simulink model "bergman_otro_modelo"  (R2019b)
settings: Solver=VariableStepAuto  StartTime=0.0  StopTime=86400  RelTol=1e-3
undefined symbols (not defined in the file): n, p1, p2, p3, Vi
libraries: simulink x16
settings Model: Creator=USUARIO  LastModifiedBy=USUARIO

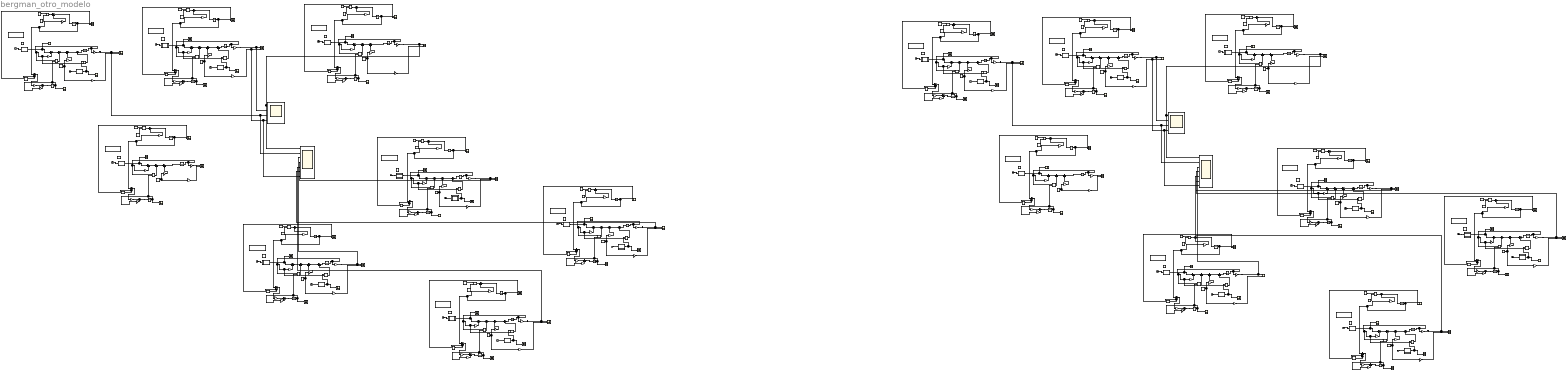
== system bergman_otro_modelo ==
  Clock{1..28} (28 alike) : Clock
  Constant{1,3,5,7,9,11,13,15,17,19,21,24,26,28,30,32} (16 alike) : Constant  Value=0
  Constant{2,4,6,8,10,12,14,16,18,20,22..23,25,27,29,31} (16 alike) : Constant  Value=Vi
  Divide{1..16} (16 alike) : Product  Inputs=*/
  Gain{1,6,11,13,18,20,25,27,32,34,39,41,46,48,50,52,54,59,62,67..68,73,76,82,84,89,92,97,99,102..103,109} (32 alike) : Gain  Gain=p1
  Gain{3,5,8,10,15,17,22,24,29,31,36,38,43,45,51,56,58,64,66,70,72,78..79,81,86,88,94,96,101,106,108,111} (32 alike) : Gain  Gain=18
  Gain{2,14,21,28,35,42,49,55,61,63,69,77,85,93,100,104} (16 alike) : Gain  Gain=p3
  Gain{7,12,19,26,33,40,47,53,60,74..75,83,91,98,105,110} (16 alike) : Gain  Gain=p2
  Gain{4,9,16,23,30,37,44,57,65,71,80,87,90,95,107,112} (16 alike) : Gain  Gain=n
  Glucosa basal{1..16} (16 alike) : Constant  Value=7
  Grafica ingesta D{1..28} (28 alike) : Scope
  Ingesta 75 g1 : MATLAB Function  TreatAsAtomicUnit=on
  Ingesta 75 g10 : MATLAB Function  TreatAsAtomicUnit=on
  Ingesta 75 g11 : MATLAB Function  TreatAsAtomicUnit=on
  Ingesta 75 g12 : MATLAB Function  TreatAsAtomicUnit=on
  Ingesta 75 g13 : MATLAB Function  TreatAsAtomicUnit=on
  Ingesta 75 g14 : MATLAB Function  TreatAsAtomicUnit=on
  Ingesta 75 g15 : MATLAB Function  TreatAsAtomicUnit=on
  Ingesta 75 g16 : MATLAB Function  TreatAsAtomicUnit=on
  Ingesta 75 g2 : MATLAB Function  TreatAsAtomicUnit=on
  Ingesta 75 g3 : MATLAB Function  TreatAsAtomicUnit=on
  Ingesta 75 g4 : MATLAB Function  TreatAsAtomicUnit=on
  Ingesta 75 g5 : MATLAB Function  TreatAsAtomicUnit=on
  Ingesta 75 g6 : MATLAB Function  TreatAsAtomicUnit=on
  Ingesta 75 g7 : MATLAB Function  TreatAsAtomicUnit=on
  Ingesta 75 g8 : MATLAB Function  TreatAsAtomicUnit=on
  Ingesta 75 g9 : MATLAB Function  TreatAsAtomicUnit=on
  Insulina basal{1..16} (16 alike) : Constant  Value=10
  Integrator{1,4,7,10,13,16,19} (7 alike) : Integrator  InitialCondition=10
  Integrator{2,5,8,11,14,17,20,24,27,30,32,36..37,41,44,47} (16 alike) : Integrator  InitialCondition=7
  Integrator{3,6,9,12,15,18,21..23,25..26,28..29,31,34..35,38..40,43,45..46,48} (23 alike) : Integrator
  Integrator33 : Integrator  InitialCondition=-0.000194
  Integrator42 : Integrator  InitialCondition=-0.000194
  MATLAB Function1 : MATLAB Function  TreatAsAtomicUnit=on
  MATLAB Function10 : MATLAB Function  TreatAsAtomicUnit=on
  MATLAB Function11 : MATLAB Function  TreatAsAtomicUnit=on
  MATLAB Function12 : MATLAB Function  TreatAsAtomicUnit=on
  MATLAB Function2 : MATLAB Function  TreatAsAtomicUnit=on
  MATLAB Function3 : MATLAB Function  TreatAsAtomicUnit=on
  MATLAB Function4 : MATLAB Function  TreatAsAtomicUnit=on
  MATLAB Function5 : MATLAB Function  TreatAsAtomicUnit=on
  MATLAB Function6 : MATLAB Function  TreatAsAtomicUnit=on
  MATLAB Function7 : MATLAB Function  TreatAsAtomicUnit=on
  MATLAB Function8 : MATLAB Function  TreatAsAtomicUnit=on
  MATLAB Function9 : MATLAB Function  TreatAsAtomicUnit=on
  Model Info1 : simulink/Model-Wide Utilities/Model Info  Frame=on  DisplayStringWithTags=|  HorizontalTextAlignment=Center  LeftAlignmentValue=0.5
      | MODELO MODIFICADO
      | 
      | INGESTA SIN INSULINA
      | 
      | PERSONA DIABETICA tipo 1
  Model Info10 : simulink/Model-Wide Utilities/Model Info  Frame=on  DisplayStringWithTags=|  HorizontalTextAlignment=Center  LeftAlignmentValue=0.5
      | MODELO MODIFICADO
      | 
      | INGESTA SIN INSULINA
      | 
      | PERSONA DIABETICA tipo 1
  Model Info11 : simulink/Model-Wide Utilities/Model Info  Frame=on  DisplayStringWithTags=|  HorizontalTextAlignment=Center  LeftAlignmentValue=0.5
      | MODELO MODIFICADO
      | 
      | INGESTA SIN INSULINA
      | 
      | PERSONA DIABETICA tipo 1
  Model Info12 : simulink/Model-Wide Utilities/Model Info  Frame=on  DisplayStringWithTags=|  HorizontalTextAlignment=Center  LeftAlignmentValue=0.5
      | MODELO MODIFICADO
      | 
      | INGESTA SIN INSULINA
      | 
      | PERSONA DIABETICA tipo 1
  Model Info13 : simulink/Model-Wide Utilities/Model Info  Frame=on  DisplayStringWithTags=|  HorizontalTextAlignment=Center  LeftAlignmentValue=0.5
      | MODELO MODIFICADO
      | 
      | TRAS INGESTA CON INSULINA
      | 
      | PERSONA DIABETICA
  Model Info14 : simulink/Model-Wide Utilities/Model Info  Frame=on  DisplayStringWithTags=|  HorizontalTextAlignment=Center  LeftAlignmentValue=0.5
      | MODELO MODIFICADO
      | 
      | INGESTA SIN INSULINA
      | 
      | PERSONA DIABETICA tipo 1
  Model Info15 : simulink/Model-Wide Utilities/Model Info  Frame=on  DisplayStringWithTags=|  HorizontalTextAlignment=Center  LeftAlignmentValue=0.5
      | MODELO MODIFICADO
      | 
      | INGESTA SIN INSULINA
      | 
      | PERSONA DIABETICA tipo 1
  Model Info16 : simulink/Model-Wide Utilities/Model Info  Frame=on  DisplayStringWithTags=|  HorizontalTextAlignment=Center  LeftAlignmentValue=0.5
      | MODELO MODIFICADO
      | 
      | INGESTA SIN INSULINA
      | 
      | PERSONA DIABETICA tipo 1
  Model Info2 : simulink/Model-Wide Utilities/Model Info  Frame=on  DisplayStringWithTags=|  HorizontalTextAlignment=Center  LeftAlignmentValue=0.5
      | MODELO MODIFICADO
      | 
      | INGESTA SIN INSULINA
      | 
      | PERSONA DIABETICA tipo 1
  Model Info3 : simulink/Model-Wide Utilities/Model Info  Frame=on  DisplayStringWithTags=|  HorizontalTextAlignment=Center  LeftAlignmentValue=0.5
      | MODELO MODIFICADO
      | 
      | INGESTA SIN INSULINA
      | 
      | PERSONA DIABETICA tipo 1
  Model Info4 : simulink/Model-Wide Utilities/Model Info  Frame=on  DisplayStringWithTags=|  HorizontalTextAlignment=Center  LeftAlignmentValue=0.5
      | MODELO MODIFICADO
      | 
      | INGESTA SIN INSULINA
      | 
      | PERSONA DIABETICA tipo 1
  Model Info5 : simulink/Model-Wide Utilities/Model Info  Frame=on  DisplayStringWithTags=|  HorizontalTextAlignment=Center  LeftAlignmentValue=0.5
      | MODELO MODIFICADO
      | 
      | INGESTA SIN INSULINA
      | 
      | PERSONA DIABETICA tipo 1
  Model Info6 : simulink/Model-Wide Utilities/Model Info  Frame=on  DisplayStringWithTags=|  HorizontalTextAlignment=Center  LeftAlignmentValue=0.5
      | MODELO MODIFICADO
      | 
      | INGESTA SIN INSULINA
      | 
      | PERSONA DIABETICA tipo 1
  Model Info7 : simulink/Model-Wide Utilities/Model Info  Frame=on  DisplayStringWithTags=|  HorizontalTextAlignment=Center  LeftAlignmentValue=0.5
      | MODELO MODIFICADO
      | 
      | INGESTA SIN INSULINA
      | 
      | PERSONA DIABETICA tipo 1
  Model Info8 : simulink/Model-Wide Utilities/Model Info  Frame=on  DisplayStringWithTags=|  HorizontalTextAlignment=Center  LeftAlignmentValue=0.5
      | MODELO MODIFICADO
      | 
      | INGESTA SIN INSULINA
      | 
      | PERSONA DIABETICA tipo 1
  Model Info9 : simulink/Model-Wide Utilities/Model Info  Frame=on  DisplayStringWithTags=|  HorizontalTextAlignment=Center  LeftAlignmentValue=0.5
      | MODELO MODIFICADO
      | 
      | TRAS INGESTA CON INSULINA
      | 
      | PERSONA DIABETICA
  Product{1..28} (28 alike) : Product
  Sum{1..2,4..12,14..19,21..26,28..33,35..40,42..47,49..52,54..60,62..66,68..73,75..76,78..81,83..89,91..96,98..101,103..108} (92 alike) : Sum  Inputs=|+-
  Sum{3,13,20,27,34,41,48,53,61,67,74,77,82,90,97,102} (16 alike) : Sum  Inputs=|++
  U (ins. exógena) cte{1..2,6,8,10,15} (6 alike) : Constant  Value=0
  U (ins. exógena) cte{7,9,11,16} (4 alike) : Constant  Value=0.185
  U (ins. exógena) cte12 : Constant  Value=0.0925
  U (ins. exógena) cte13 : Constant  Value=0.06167
  U (ins. exógena) cte14 : Constant  Value=0.1233
  U (ins. exógena) cte3 : Constant  Value=0.0925
  U (ins. exógena) cte4 : Constant  Value=0.06167
  U (ins. exógena) cte5 : Constant  Value=0.1233
  glucosa tras ingesta1 : Scope  NumInputPorts=4
  glucosa tras ingesta{2..3,5..10,12..14,16..20} (16 alike) : Scope  NumInputPorts=2
  glucosa tras ingesta11 : Scope  NumInputPorts=4
  glucosa tras ingesta15 : Scope  NumInputPorts=7
  glucosa tras ingesta4 : Scope  NumInputPorts=7
  grafica insulina{1..16} (16 alike) : Scope  NumInputPorts=2
  insulina activa{1..16} (16 alike) : Scope
  wires:
  Sum38/1 -> Integrator17/1
  Clock12/1 -> Ingesta 75 g6/1(in)
  Divide6/1 -> Sum37/1
  Sum35/1 -> Integrator18/1
  U (ins. exógena) cte6/1 -> Divide6/1
  Gain41/1 -> Sum40/2
  Constant12/1 -> Divide6/2
  MATLAB Function4/1(Ej) -> Product13/1, Grafica ingesta D13/1
  Sum37/1 -> Integrator16/1
  Insulina basal6/1 -> grafica insulina6/2, Sum39/2  "insulina basal"
  Gain36/1 -> glucosa tras ingesta1/2, glucosa tras ingesta7/1  "Ejercicio previo a la ingesta: Periodo corto"
  Gain39/1 -> Sum41/2
  Ingesta 75 g6/1(D) -> Grafica ingesta D12/1, Sum40/1
  Integrator17/1 -> Gain36/1, Product12/1, Product13/2, Gain41/1  "G(t)"
  Product12/1 -> Sum36/2
  Sum36/1 -> Sum41/1
  Gain38/1 -> glucosa tras ingesta4/7, glucosa tras ingesta1/4, glucosa tras ingesta7/2  "glucosa basal diabetico"
  Integrator16/1 -> grafica insulina6/1, Gain37/1, Sum39/1  "I(t)"
  Gain37/1 -> Sum37/2
  Glucosa basal6/1 -> Gain39/1, Gain38/1  "glucosa basal"
  Sum41/1 -> Sum38/1
  Gain40/1 -> Sum35/2
  Gain42/1 -> Sum35/1
  Integrator18/1 -> insulina activa6/1, Product12/2, Gain40/1  "X(t)"
  Clock9/1 -> MATLAB Function4/1(in)
  Sum40/1 -> Sum36/1
  Product13/1 -> Sum38/2
  Sum39/1 -> Gain42/1
  Sum3/1 -> Integrator2/1
  Sum2/1 -> Sum5/1
  Gain2/1 -> Sum4/1
  Sum6/1 -> Integrator1/1
  Integrator1/1 -> grafica insulina1/1, Gain4/1, Sum1/1  "I(t)"
  Integrator2/1 -> Gain3/1, Product1/1, Gain1/1  "G(t)"
  Gain1/1 -> Sum2/2
  U (ins. exógena) cte1/1 -> Divide1/1
  Clock1/1 -> Ingesta 75 g1/1(in)
  Product1/1 -> Sum5/2
  Constant2/1 -> Divide1/2
  Gain4/1 -> Sum6/2
  Divide1/1 -> Sum6/1
  Gain6/1 -> Sum3/2
  Sum4/1 -> Integrator3/1
  Gain5/1 -> glucosa tras ingesta2/2  "glucosa basal diabetico"
  Gain3/1 -> glucosa tras ingesta1/1, glucosa tras ingesta4/1, glucosa tras ingesta2/1  "Ingesta"
  Integrator3/1 -> insulina activa1/1, Product1/2, Gain7/1  "X(t)"
  Sum5/1 -> Sum3/1
  Insulina basal1/1 -> grafica insulina1/2, Sum1/2  "insulina basal"
  Ingesta 75 g1/1(D) -> Grafica ingesta D1/1, Sum2/1
  Sum1/1 -> Gain2/1
  Glucosa basal1/1 -> Gain6/1, Gain5/1  "glucosa basal"
  Gain7/1 -> Sum4/2
  Divide11/1 -> Sum64/1
  Gain72/1 -> glucosa tras ingesta10/2  "glucosa basal"
  Integrator32/1 -> Gain70/1, Product11/1, Gain68/1  "G(t)"
  Sum62/1 -> Integrator33/1
  Gain70/1 -> glucosa tras ingesta10/1  "Ingesta con insulina"
  U (ins. exógena) cte11/1 -> Divide11/1
  Sum59/1 -> Gain69/1
  Insulina basal11/1 -> grafica insulina12/2, Sum59/2  "insulina basal"
  Sum63/1 -> Sum61/1
  Gain73/1 -> Sum61/2
  Sum61/1 -> Integrator32/1
  Sum60/1 -> Sum63/1
  Clock11/1 -> Ingesta 75 g11/1(in)
  Integrator33/1 -> insulina activa11/1, Product11/2, Gain74/1  "X(t)"
  Integrator31/1 -> grafica insulina12/1, Gain71/1, Sum59/1  "I(t)"
  Sum64/1 -> Integrator31/1
  Constant22/1 -> Divide11/2
  Gain69/1 -> Sum62/1
  Gain74/1 -> Sum62/2
  Glucosa basal11/1 -> Gain73/1, Gain72/1  "glucosa basal"
  Ingesta 75 g11/1(D) -> Grafica ingesta D11/1, Sum60/1
  Product11/1 -> Sum63/2
  Gain71/1 -> Sum64/2
  Gain68/1 -> Sum60/2
  Insulina basal2/1 -> grafica insulina2/2, Sum11/2  "insulina basal"
  Gain8/1 -> glucosa tras ingesta4/2, glucosa tras ingesta1/3, glucosa tras ingesta3/1  "Ejercicio tras ingesta: Periodo corto"
  MATLAB Function1/1(Ej) -> Product3/1, Grafica ingesta D3/1
  Sum9/1 -> Integrator4/1
  U (ins. exógena) cte2/1 -> Divide2/1
  Clock2/1 -> Ingesta 75 g2/1(in)
  Constant4/1 -> Divide2/2
  Sum10/1 -> Integrator5/1
  Sum11/1 -> Gain14/1
  Divide2/1 -> Sum9/1
  Sum12/1 -> Sum8/1
  Integrator6/1 -> insulina activa2/1, Product2/2, Gain12/1  "X(t)"
  Gain14/1 -> Sum7/1
  Glucosa basal2/1 -> Gain11/1, Gain10/1  "glucosa basal"
  Gain9/1 -> Sum9/2
  Gain12/1 -> Sum7/2
  Gain10/1 -> glucosa tras ingesta3/2  "glucosa basal diabetico"
  Integrator4/1 -> grafica insulina2/1, Gain9/1, Sum11/1  "I(t)"
  Sum8/1 -> Sum13/1
  Product2/1 -> Sum8/2
  Ingesta 75 g2/1(D) -> Grafica ingesta D2/1, Sum12/1
  Gain11/1 -> Sum13/2
  Clock3/1 -> MATLAB Function1/1(in)
  Gain13/1 -> Sum12/2
  Integrator5/1 -> Gain8/1, Product2/1, Product3/2, Gain13/1  "G(t)"
  Sum7/1 -> Integrator6/1
  Sum13/1 -> Sum10/1
  Product3/1 -> Sum10/2
  Insulina basal3/1 -> grafica insulina3/2, Sum18/2  "insulina basal"
  Gain15/1 -> glucosa tras ingesta4/4, glucosa tras ingesta5/1  "Ejercicio con insulina: 1/2 dosis original"
  MATLAB Function2/1(Ej) -> Product5/1, Grafica ingesta D5/1
  Sum16/1 -> Integrator7/1
  U (ins. exógena) cte3/1 -> Divide3/1
  Clock4/1 -> Ingesta 75 g3/1(in)
  Sum17/1 -> Integrator8/1
  Sum18/1 -> Gain21/1
  Divide3/1 -> Sum16/1
  Sum19/1 -> Sum15/1
  Integrator9/1 -> insulina activa3/1, Product4/2, Gain19/1  "X(t)"
  Gain21/1 -> Sum14/1
  Glucosa basal3/1 -> Gain18/1, Gain17/1  "glucosa basal"
  Gain16/1 -> Sum16/2
  Gain19/1 -> Sum14/2
  Gain17/1 -> glucosa tras ingesta5/2  "glucosa basal diabetico"
  Integrator7/1 -> grafica insulina3/1, Gain16/1, Sum18/1  "I(t)"
  Sum15/1 -> Sum20/1
  Product4/1 -> Sum15/2
  Gain18/1 -> Sum20/2
  Clock5/1 -> MATLAB Function2/1(in)
  Gain20/1 -> Sum19/2
  Integrator8/1 -> Gain15/1, Product4/1, Product5/2, Gain20/1  "G(t)"
  Sum14/1 -> Integrator9/1
  Sum20/1 -> Sum17/1
  Ingesta 75 g3/1(D) -> Grafica ingesta D4/1, Sum19/1
  Product5/1 -> Sum17/2
  Constant6/1 -> Divide3/2
  Insulina basal4/1 -> grafica insulina4/2, Sum25/2  "insulina basal"
  Gain22/1 -> glucosa tras ingesta4/3, glucosa tras ingesta6/1  "Ejercicio con insulina: 1/3 dosis original"
  MATLAB Function3/1(Ej) -> Product7/1, Grafica ingesta D7/1
  Sum23/1 -> Integrator10/1
  U (ins. exógena) cte4/1 -> Divide4/1
  Clock6/1 -> Ingesta 75 g4/1(in)
  Sum24/1 -> Integrator11/1
  Sum25/1 -> Gain28/1
  Divide4/1 -> Sum23/1
  Sum26/1 -> Sum22/1
  Integrator12/1 -> insulina activa4/1, Product6/2, Gain26/1  "X(t)"
  Gain28/1 -> Sum21/1
  Glucosa basal4/1 -> Gain25/1, Gain24/1  "glucosa basal"
  Gain23/1 -> Sum23/2
  Gain26/1 -> Sum21/2
  Gain24/1 -> glucosa tras ingesta6/2  "glucosa basal diabetico"
  Integrator10/1 -> grafica insulina4/1, Gain23/1, Sum25/1  "I(t)"
  Sum22/1 -> Sum27/1
  Product6/1 -> Sum22/2
  Gain25/1 -> Sum27/2
  Clock7/1 -> MATLAB Function3/1(in)
  Gain27/1 -> Sum26/2
  Integrator11/1 -> Gain22/1, Product6/1, Product7/2, Gain27/1  "G(t)"
  Sum21/1 -> Integrator12/1
  Sum27/1 -> Sum24/1
  Ingesta 75 g4/1(D) -> Grafica ingesta D6/1, Sum26/1
  Product7/1 -> Sum24/2
  Constant8/1 -> Divide4/2
  Gain34/1 -> Sum33/2
  Clock10/1 -> MATLAB Function5/1(in)
  Product8/1 -> Sum29/2
  Gain32/1 -> Sum34/2
  Integrator13/1 -> grafica insulina5/1, Gain30/1, Sum32/1  "I(t)"
  Sum31/1 -> Integrator14/1
  Clock8/1 -> Ingesta 75 g5/1(in)
  U (ins. exógena) cte5/1 -> Divide5/1
  Sum30/1 -> Integrator13/1
  MATLAB Function5/1(Ej) -> Product9/1, Grafica ingesta D9/1
  Insulina basal5/1 -> grafica insulina5/2, Sum32/2  "insulina basal"
  Ingesta 75 g5/1(D) -> Grafica ingesta D8/1, Sum33/1
  Constant10/1 -> Divide5/2
  Product9/1 -> Sum31/2
  Sum28/1 -> Integrator15/1
  Integrator14/1 -> Gain29/1, Product8/1, Product9/2, Gain34/1  "G(t)"
  Sum32/1 -> Gain35/1
  Sum29/1 -> Sum34/1
  Sum34/1 -> Sum31/1
  Integrator15/1 -> insulina activa5/1, Product8/2, Gain33/1  "X(t)"
  Gain31/1 -> glucosa tras ingesta8/2  "glucosa basal diabetico"
  Gain33/1 -> Sum28/2
  Gain29/1 -> glucosa tras ingesta4/5, glucosa tras ingesta8/1  "Ejercicio con insulina: 2/3 dosis original"
  Glucosa basal5/1 -> Gain32/1, Gain31/1  "glucosa basal"
  Gain35/1 -> Sum28/1
  Gain30/1 -> Sum30/2
  Divide5/1 -> Sum30/1
  Sum33/1 -> Sum29/1
  Gain48/1 -> Sum47/2
  Clock14/1 -> MATLAB Function6/1(in)
  Product10/1 -> Sum43/2
  Gain46/1 -> Sum48/2
  Integrator19/1 -> grafica insulina7/1, Gain44/1, Sum46/1  "I(t)"
  Sum45/1 -> Integrator20/1
  Clock13/1 -> Ingesta 75 g7/1(in)
  U (ins. exógena) cte7/1 -> Divide7/1
  Sum44/1 -> Integrator19/1
  MATLAB Function6/1(Ej) -> Product14/1, Grafica ingesta D14/1
  Insulina basal7/1 -> grafica insulina7/2, Sum46/2  "insulina basal"
  Ingesta 75 g7/1(D) -> Grafica ingesta D10/1, Sum47/1
  Constant14/1 -> Divide7/2
  Product14/1 -> Sum45/2
  Sum42/1 -> Integrator21/1
  Integrator20/1 -> Gain43/1, Product10/1, Product14/2, Gain48/1  "G(t)"
  Sum46/1 -> Gain49/1
  Sum43/1 -> Sum48/1
  Sum48/1 -> Sum45/1
  Integrator21/1 -> insulina activa7/1, Product10/2, Gain47/1  "X(t)"
  Gain45/1 -> glucosa tras ingesta9/2  "glucosa basal diabetico"
  Gain47/1 -> Sum42/2
  Gain43/1 -> glucosa tras ingesta4/6, glucosa tras ingesta9/1  "Ejercicio con insulina: dosis original"
  Glucosa basal7/1 -> Gain46/1, Gain45/1  "glucosa basal"
  Gain49/1 -> Sum42/1
  Gain44/1 -> Sum44/2
  Divide7/1 -> Sum44/1
  Sum47/1 -> Sum43/1
  U (ins. exógena) cte9/1 -> Divide9/1
  U (ins. exógena) cte12/1 -> Divide12/1
  Integrator23/1 -> grafica insulina13/1, Gain65/1, Sum72/1  "I(t)"
  Integrator47/1 -> Gain56/1, Product23/1, Product24/2, Gain62/1  "G(t)"
  U (ins. exógena) cte10/1 -> Divide10/1
  Insulina basal15/1 -> grafica insulina15/2, Sum87/2  "insulina basal"
  Gain86/1 -> glucosa tras ingesta11/2, glucosa tras ingesta18/1  "Ejercicio previo a la ingesta: Periodo medio"
  Clock26/1 -> MATLAB Function9/1(in)
  Sum85/1 -> Integrator29/1
  Clock18/1 -> Ingesta 75 g15/1(in)
  Sum83/1 -> Integrator34/1
  Sum87/1 -> Gain93/1
  Clock28/1 -> MATLAB Function10/1(in)
  Integrator34/1 -> insulina activa15/1, Product18/2, Gain91/1  "X(t)"
  Glucosa basal15/1 -> Gain89/1, Gain88/1  "glucosa basal"
  Gain88/1 -> glucosa tras ingesta15/7, glucosa tras ingesta11/4, glucosa tras ingesta18/2  "glucosa basal diabetico"
  Product18/1 -> Sum84/2
  Product25/1 -> Sum69/2
  Sum84/1 -> Sum90/1
  Gain89/1 -> Sum90/2
  Integrator30/1 -> Gain86/1, Product18/1, Product19/2, Gain92/1  "G(t)"
  Sum98/1 -> Sum77/1
  Gain90/1 -> Sum100/2
  Constant23/1 -> Divide8/2
  Product15/1 -> Sum98/2
  U (ins. exógena) cte8/1 -> Divide8/1
  Clock15/1 -> Ingesta 75 g8/1(in)
  Sum66/1 -> Sum98/1
  Gain61/1 -> Sum88/1
  Sum77/1 -> Integrator36/1
  Divide16/1 -> Sum93/1
  Gain80/1 -> Sum78/2
  Gain87/1 -> Sum85/2
  Sum81/1 -> Sum76/1
  Gain85/1 -> Sum75/1
  Glucosa basal14/1 -> Gain82/1, Gain81/1  "glucosa basal"
  Gain67/1 -> Sum74/2
  Sum76/1 -> Sum82/1
  Sum96/1 -> Sum92/1
  Product28/1 -> Sum79/2
  Integrator27/1 -> Gain78/1, Product27/1, Product28/2, Gain84/1  "G(t)"
  Ingesta 75 g15/1(D) -> Grafica ingesta D18/1, Sum89/1
  Integrator39/1 -> insulina activa8/1, Product15/2, Gain105/1  "X(t)"
  Sum75/1 -> Integrator28/1
  Constant16/1 -> Divide14/2
  Ingesta 75 g14/1(D) -> Grafica ingesta D27/1, Sum81/1
  MATLAB Function11/1(Ej) -> Product28/1, Grafica ingesta D28/1
  Insulina basal14/1 -> grafica insulina14/2, Sum80/2  "insulina basal"
  Sum79/1 -> Integrator27/1
  Clock16/1 -> MATLAB Function11/1(in)
  Gain84/1 -> Sum81/2
  Sum72/1 -> Gain77/1
  MATLAB Function7/1(Ej) -> Product22/1, Grafica ingesta D22/1
  Divide15/1 -> Sum85/1
  Integrator29/1 -> grafica insulina15/1, Gain87/1, Sum87/1  "I(t)"
  Sum70/1 -> Integrator23/1
  MATLAB Function9/1(Ej) -> Product26/1, Grafica ingesta D26/1
  Constant18/1 -> Divide15/2
  Integrator26/1 -> grafica insulina14/1, Gain80/1, Sum80/1  "I(t)"
  Divide8/1 -> Sum100/1
  Product17/1 -> Sum104/2
  Sum56/1 -> Integrator46/1
  Gain103/1 -> Sum101/2
  Sum105/1 -> Integrator40/1
  Sum90/1 -> Sum86/1
  Sum101/1 -> Sum104/1
  Sum102/1 -> Integrator41/1
  Insulina basal9/1 -> grafica insulina9/2, Sum99/2  "insulina basal"
  U (ins. exógena) cte13/1 -> Divide13/1
  Constant25/1 -> Divide9/2
  Gain110/1 -> Sum103/2
  Gain104/1 -> Sum103/1
  Glucosa basal8/1 -> Gain102/1, Gain101/1  "glucosa basal"
  Gain105/1 -> Sum88/2
  Ingesta 75 g8/1(D) -> Grafica ingesta D15/1, Sum66/1
  Sum49/1 -> Gain61/1
  Divide14/1 -> Sum78/1
  Integrator42/1 -> insulina activa9/1, Product17/2, Gain110/1  "X(t)"
  Sum69/1 -> Sum74/1
  Sum99/1 -> Gain104/1
  Sum67/1 -> Sum57/1
  Gain106/1 -> glucosa tras ingesta12/1  "Ingesta con insulina"
  Clock21/1 -> Ingesta 75 g10/1(in)
  Sum51/1 -> Gain55/1
  Sum100/1 -> Integrator22/1
  Sum104/1 -> Sum102/1
  Gain111/1 -> glucosa tras ingesta15/2, glucosa tras ingesta11/3, glucosa tras ingesta14/1  "Ejercicio tras ingesta: Periodo medio"
  Sum82/1 -> Sum79/1
  U (ins. exógena) cte15/1 -> Divide15/1
  Insulina basal13/1 -> grafica insulina13/2, Sum72/2  "insulina basal"
  Gain50/1 -> Sum66/2
  Ingesta 75 g13/1(D) -> Grafica ingesta D25/1, Sum73/1
  Gain64/1 -> glucosa tras ingesta15/3, glucosa tras ingesta17/1  "Ejercicio con insulina: 1/3 dosis original"
  Constant31/1 -> Divide13/2
  Product26/1 -> Sum71/2
  Gain101/1 -> glucosa tras ingesta13/2  "glucosa basal diabetico"
  Constant29/1 -> Divide12/2
  Sum108/1 -> Integrator43/1
  Product22/1 -> Sum50/2
  Sum106/1 -> Integrator45/1
  Sum53/1 -> Sum50/1
  Glucosa basal9/1 -> Gain109/1, Gain108/1  "glucosa basal"
  Gain108/1 -> glucosa tras ingesta12/2  "glucosa basal"
  Ingesta 75 g12/1(D) -> Grafica ingesta D23/1, Sum65/1
  Sum86/1 -> Integrator30/1
  MATLAB Function12/1(Ej) -> Product20/1, Grafica ingesta D20/1
  Product19/1 -> Sum86/2
  Insulina basal12/1 -> grafica insulina11/2, Sum58/2  "insulina basal"
  Sum93/1 -> Integrator35/1
  U (ins. exógena) cte14/1 -> Divide14/1
  Clock19/1 -> Ingesta 75 g16/1(in)
  Sum94/1 -> Integrator37/1
  Gain97/1 -> Sum97/2
  Integrator40/1 -> grafica insulina9/1, Gain107/1, Sum99/1  "I(t)"
  Gain91/1 -> Sum83/2
  Integrator35/1 -> grafica insulina16/1, Gain95/1, Sum95/1  "I(t)"
  Sum54/1 -> Integrator48/1
  U (ins. exógena) cte16/1 -> Divide16/1
  Clock20/1 -> MATLAB Function12/1(in)
  Gain100/1 -> Sum91/1
  Gain94/1 -> glucosa tras ingesta15/6, glucosa tras ingesta20/1  "Ejercicio con insulina: dosis original"
  Product27/1 -> Sum76/2
  Sum92/1 -> Sum97/1
  Sum97/1 -> Sum94/1
  Insulina basal16/1 -> grafica insulina16/2, Sum95/2  "insulina basal"
  Integrator38/1 -> insulina activa16/1, Product16/2, Gain98/1  "X(t)"
  Sum95/1 -> Gain100/1
  Integrator37/1 -> Gain94/1, Product16/1, Product20/2, Gain99/1  "G(t)"
  Gain102/1 -> Sum77/2
  Insulina basal8/1 -> grafica insulina8/2, Sum49/2  "insulina basal"
  Product20/1 -> Sum94/2
  Ingesta 75 g16/1(D) -> Grafica ingesta D16/1, Sum96/1
  Gain95/1 -> Sum93/2
  Constant20/1 -> Divide16/2
  Sum107/1 -> Sum53/1
  Integrator43/1 -> grafica insulina10/1, Gain112/1, Sum51/1  "I(t)"
  Gain51/1 -> glucosa tras ingesta14/2  "glucosa basal diabetico"
  Product16/1 -> Sum92/2
  Sum71/1 -> Integrator24/1
  Gain82/1 -> Sum82/2
  Gain53/1 -> Sum106/2
  Gain109/1 -> Sum102/2
  Sum80/1 -> Gain85/1
  Gain112/1 -> Sum108/2
  Sum78/1 -> Integrator26/1
  Gain55/1 -> Sum106/1
  Integrator45/1 -> insulina activa10/1, Product21/2, Gain53/1  "X(t)"
  Glucosa basal10/1 -> Gain52/1, Gain51/1  "glucosa basal"
  Gain99/1 -> Sum96/2
  Sum52/1 -> Sum107/1
  Divide10/1 -> Sum108/1
  Gain96/1 -> glucosa tras ingesta20/2  "glucosa basal diabetico"
  Integrator36/1 -> Gain79/1, Product15/1, Gain50/1  "G(t)"
  Product21/1 -> Sum107/2
  Gain78/1 -> glucosa tras ingesta15/5, glucosa tras ingesta19/1  "Ejercicio con insulina: 2/3 dosis original"
  Integrator41/1 -> Gain106/1, Product17/1, Gain103/1  "G(t)"
  Sum103/1 -> Integrator42/1
  Divide9/1 -> Sum105/1
  Gain54/1 -> Sum52/2
  Gain81/1 -> glucosa tras ingesta19/2  "glucosa basal diabetico"
  Insulina basal10/1 -> grafica insulina10/2, Sum51/2  "insulina basal"
  Gain98/1 -> Sum91/2
  Constant27/1 -> Divide10/2
  Gain58/1 -> glucosa tras ingesta16/2  "glucosa basal diabetico"
  Sum68/1 -> Integrator25/1
  Integrator48/1 -> insulina activa12/1, Product23/2, Gain60/1  "X(t)"
  Clock25/1 -> Ingesta 75 g13/1(in)
  Clock27/1 -> Ingesta 75 g14/1(in)
  Gain57/1 -> Sum56/2
  MATLAB Function10/1(Ej) -> Product19/1, Grafica ingesta D19/1
  Glucosa basal16/1 -> Gain97/1, Gain96/1  "glucosa basal"
  Divide12/1 -> Sum56/1
  Gain92/1 -> Sum89/2
  Clock23/1 -> Ingesta 75 g12/1(in)
  Integrator24/1 -> Gain64/1, Product25/1, Product26/2, Gain76/1  "G(t)"
  Gain62/1 -> Sum65/2
  Integrator44/1 -> Gain111/1, Product21/1, Product22/2, Gain54/1  "G(t)"
  Gain76/1 -> Sum73/2
  Sum91/1 -> Integrator38/1
  Gain107/1 -> Sum105/2
  Clock24/1 -> MATLAB Function8/1(in)
  Clock17/1 -> Ingesta 75 g9/1(in)
  Product23/1 -> Sum55/2
  Sum55/1 -> Sum67/1
  Sum74/1 -> Sum71/1
  Sum58/1 -> Gain63/1
  Integrator28/1 -> insulina activa14/1, Product27/2, Gain83/1  "X(t)"
  Ingesta 75 g9/1(D) -> Grafica ingesta D17/1, Sum101/1
  Gain93/1 -> Sum83/1
  Gain63/1 -> Sum54/1
  Glucosa basal12/1 -> Gain59/1, Gain58/1  "glucosa basal"
  Integrator25/1 -> insulina activa13/1, Product25/2, Gain75/1  "X(t)"
  Sum89/1 -> Sum84/1
  Integrator46/1 -> grafica insulina11/1, Gain57/1, Sum58/1  "I(t)"
  Gain75/1 -> Sum68/2
  Gain65/1 -> Sum70/2
  Sum65/1 -> Sum55/1
  Product24/1 -> Sum57/2
  Gain77/1 -> Sum68/1
  Gain60/1 -> Sum54/2
  Sum88/1 -> Integrator39/1
  Sum50/1 -> Integrator44/1
  Gain59/1 -> Sum67/2
  Divide13/1 -> Sum70/1
  Gain83/1 -> Sum75/2
  Ingesta 75 g10/1(D) -> Grafica ingesta D21/1, Sum52/1
  Gain79/1 -> glucosa tras ingesta11/1, glucosa tras ingesta15/1, glucosa tras ingesta13/1  "Ingesta"
  Sum57/1 -> Integrator47/1
  MATLAB Function8/1(Ej) -> Product24/1, Grafica ingesta D24/1
  Sum73/1 -> Sum69/1
  Gain52/1 -> Sum53/2
  Gain56/1 -> glucosa tras ingesta15/4, glucosa tras ingesta16/1  "Ejercicio con insulina: 1/2 dosis original"
  Gain66/1 -> glucosa tras ingesta17/2  "glucosa basal diabetico"
  Glucosa basal13/1 -> Gain67/1, Gain66/1  "glucosa basal"
  Clock22/1 -> MATLAB Function7/1(in)
  Integrator22/1 -> grafica insulina8/1, Gain90/1, Sum49/1  "I(t)"

== matlab function bergman_otro_modelo/Ingesta 75 g1 ==
  data: in input; D output
function D = comida(in)
% Variables de entrada en la funcion
t = in(1) %- 8*60*60; % Ajuste para iniciar a las 8 de la mañana
 
% Parámetros del modelo
Ag = 0.8; % adimensional
Tmaxi = 55*60; % s
Vg = 13.79; % L
Tmaxg = 40*60; % s
t1 = 0;
Dg = 0;
f = 1000/180; % factor de conversión de g a mmol
 
% Comidas (perturbaciones) a lo largo de un día
if t >= 180*60 && t < 480*60 % ingesta de 75 g de HC
    t1 = 180*60;
    Dg = 50*f;
end
 
% Ecuación
D = (Dg*Ag*(t-t1)*exp(-(t-t1)/Tmaxi))/(Vg*Tmaxg^2);

== matlab function bergman_otro_modelo/Ingesta 75 g2 ==
  data: in input; D output
function D = comida(in)
% Variables de entrada en la funcion
t = in(1) %- 8*60*60; % Ajuste para iniciar a las 8 de la mañana
 
% Parámetros del modelo
Ag = 0.8; % adimensional
Tmaxi = 55*60; % s
Vg = 13.79; % L
Tmaxg = 40*60; % s
t1 = 0;
Dg = 0;
f = 1000/180; % factor de conversión de g a mmol
 
% Comidas (perturbaciones) a lo largo de un día
if t >= 180*60 && t < 480*60 % ingesta de 75 g de HC
    t1 = 180*60;
    Dg = 50*f;
end
 
% Ecuación
D = (Dg*Ag*(t-t1)*exp(-(t-t1)/Tmaxi))/(Vg*Tmaxg^2);

== matlab function bergman_otro_modelo/MATLAB Function1 ==
  data: in input; Ej output
function Ej  = ejercicio(in)
% Variables de entrada en la funcion
t = in(1);
%Parametros del modelo
cons = 0.005/60;
%Ejercicio (perturbaciones) a lo largo de un día

if t>=0 && t<240*60 %ejercicio 1 h
 Ej=0;
elseif t>=240*60 && t<300*60 %ejercicio 1 h
 Ej=cons+ 0.005/60;
else
 Ej=cons/4;
end

== matlab function bergman_otro_modelo/Ingesta 75 g3 ==
  data: in input; D output
function D = comida(in)
% Variables de entrada en la funcion
t = in(1) %- 8*60*60; % Ajuste para iniciar a las 8 de la mañana
 
% Parámetros del modelo
Ag = 0.8; % adimensional
Tmaxi = 55*60; % s
Vg = 13.79; % L
Tmaxg = 40*60; % s
t1 = 0;
Dg = 0;
f = 1000/180; % factor de conversión de g a mmol
 
% Comidas (perturbaciones) a lo largo de un día
if t >= 180*60 && t < 480*60 % ingesta de 75 g de HC
    t1 = 180*60;
    Dg = 50*f;
end
 
% Ecuación
D = (Dg*Ag*(t-t1)*exp(-(t-t1)/Tmaxi))/(Vg*Tmaxg^2);

== matlab function bergman_otro_modelo/MATLAB Function2 ==
  data: in input; Ej output
function Ej  = ejercicio(in)
% Variables de entrada en la funcion
t = in(1);
%Parametros del modelo
cons = 0.005/60;
%Ejercicio (perturbaciones) a lo largo de un día

if t>=0 && t<240*60 %ejercicio 1 h
 Ej=0;
elseif t>=240*60 && t<300*60 %ejercicio 1 h
 Ej=cons+ 0.005/60;
else
 Ej=cons/4;
end

== matlab function bergman_otro_modelo/Ingesta 75 g4 ==
  data: in input; D output
function D = comida(in)
% Variables de entrada en la funcion
t = in(1) %- 8*60*60; % Ajuste para iniciar a las 8 de la mañana
 
% Parámetros del modelo
Ag = 0.8; % adimensional
Tmaxi = 55*60; % s
Vg = 13.79; % L
Tmaxg = 40*60; % s
t1 = 0;
Dg = 0;
f = 1000/180; % factor de conversión de g a mmol
 
% Comidas (perturbaciones) a lo largo de un día
if t >= 180*60 && t < 480*60 % ingesta de 75 g de HC
    t1 = 180*60;
    Dg = 50*f;
end
 
% Ecuación
D = (Dg*Ag*(t-t1)*exp(-(t-t1)/Tmaxi))/(Vg*Tmaxg^2);

== matlab function bergman_otro_modelo/MATLAB Function3 ==
  data: in input; Ej output
function Ej  = ejercicio(in)
% Variables de entrada en la funcion
t = in(1);
%Parametros del modelo
cons = 0.005/60;
%Ejercicio (perturbaciones) a lo largo de un día

if t>=0 && t<240*60 %ejercicio 1 h
 Ej=0;
elseif t>=240*60 && t<300*60 %ejercicio 1 h
 Ej=cons+ 0.005/60;
else
 Ej=cons/4;
end

== matlab function bergman_otro_modelo/Ingesta 75 g5 ==
  data: in input; D output
function D = comida(in)
% Variables de entrada en la funcion
t = in(1) %- 8*60*60; % Ajuste para iniciar a las 8 de la mañana
 
% Parámetros del modelo
Ag = 0.8; % adimensional
Tmaxi = 55*60; % s
Vg = 13.79; % L
Tmaxg = 40*60; % s
t1 = 0;
Dg = 0;
f = 1000/180; % factor de conversión de g a mmol
 
% Comidas (perturbaciones) a lo largo de un día
if t >= 180*60 && t < 480*60 % ingesta de 75 g de HC
    t1 = 180*60;
    Dg = 50*f;
end
 
% Ecuación
D = (Dg*Ag*(t-t1)*exp(-(t-t1)/Tmaxi))/(Vg*Tmaxg^2);

== matlab function bergman_otro_modelo/MATLAB Function5 ==
  data: in input; Ej output
function Ej  = ejercicio(in)
% Variables de entrada en la funcion
t = in(1);
%Parametros del modelo
cons = 0.005/60;
%Ejercicio (perturbaciones) a lo largo de un día

if t>=0 && t<240*60 %ejercicio 1 h
 Ej=0;
elseif t>=240*60 && t<300*60 %ejercicio 1 h
 Ej=cons+ 0.005/60;
else
 Ej=cons/4;
end

== matlab function bergman_otro_modelo/Ingesta 75 g7 ==
  data: in input; D output
function D = comida(in)
% Variables de entrada en la funcion
t = in(1) %- 8*60*60; % Ajuste para iniciar a las 8 de la mañana
 
% Parámetros del modelo
Ag = 0.8; % adimensional
Tmaxi = 55*60; % s
Vg = 13.79; % L
Tmaxg = 40*60; % s
t1 = 0;
Dg = 0;
f = 1000/180; % factor de conversión de g a mmol
 
% Comidas (perturbaciones) a lo largo de un día
if t >= 180*60 && t < 480*60 % ingesta de 75 g de HC
    t1 = 180*60;
    Dg = 50*f;
end
 
% Ecuación
D = (Dg*Ag*(t-t1)*exp(-(t-t1)/Tmaxi))/(Vg*Tmaxg^2);

== matlab function bergman_otro_modelo/Ingesta 75 g11 ==
  data: in input; D output
function D = comida(in)
% Variables de entrada en la funcion
t = in(1) %- 8*60*60; % Ajuste para iniciar a las 8 de la mañana
 
% Parámetros del modelo
Ag = 0.8; % adimensional
Tmaxi = 55*60; % s
Vg = 13.79; % L
Tmaxg = 40*60; % s
t1 = 0;
Dg = 0;
f = 1000/180; % factor de conversión de g a mmol
 
% Comidas (perturbaciones) a lo largo de un día
if t >= 180*60 && t < 480*60 % ingesta de 75 g de HC
    t1 = 180*60;
    Dg = 50*f;
end
 
% Ecuación
D = (Dg*Ag*(t-t1)*exp(-(t-t1)/Tmaxi))/(Vg*Tmaxg^2);

== matlab function bergman_otro_modelo/Ingesta 75 g6 ==
  data: in input; D output
function D = comida(in)
% Variables de entrada en la funcion
t = in(1) %- 8*60*60; % Ajuste para iniciar a las 8 de la mañana
 
% Parámetros del modelo
Ag = 0.8; % adimensional
Tmaxi = 55*60; % s
Vg = 13.79; % L
Tmaxg = 40*60; % s
t1 = 0;
Dg = 0;
f = 1000/180; % factor de conversión de g a mmol
 
% Comidas (perturbaciones) a lo largo de un día
if t >= 180*60 && t < 480*60 % ingesta de 75 g de HC
    t1 = 180*60;
    Dg = 50*f;
end
 
% Ecuación
D = (Dg*Ag*(t-t1)*exp(-(t-t1)/Tmaxi))/(Vg*Tmaxg^2);

== matlab function bergman_otro_modelo/MATLAB Function4 ==
  data: in input; Ej output
function Ej  = ejercicio(in)
% Variables de entrada en la funcion
t = in(1);
%Parametros del modelo
cons = 0.005/60;
%Ejercicio (perturbaciones) a lo largo de un día

if t>=0 && t<120*60 %ejercicio 1 h
 Ej=0;
elseif t>=120*60 && t<180*60 %ejercicio 1 h
 Ej=cons+ 0.005/60;
else
 Ej=cons/4;
end

== matlab function bergman_otro_modelo/MATLAB Function6 ==
  data: in input; Ej output
function Ej  = ejercicio(in)
% Variables de entrada en la funcion
t = in(1);
%Parametros del modelo
cons = 0.005/60;
%Ejercicio (perturbaciones) a lo largo de un día

if t>=0 && t<240*60 %ejercicio 1 h
 Ej=0;
elseif t>=240*60 && t<300*60 %ejercicio 1 h
 Ej=cons+ 0.005/60;
else
 Ej=cons/4;
end

== matlab function bergman_otro_modelo/Ingesta 75 g10 ==
  data: in input; D output
function D = comida(in)
% Variables de entrada en la funcion
t = in(1) %- 8*60*60; % Ajuste para iniciar a las 8 de la mañana
 
% Parámetros del modelo
Ag = 0.8; % adimensional
Tmaxi = 55*60; % s
Vg = 13.79; % L
Tmaxg = 40*60; % s
t1 = 0;
Dg = 0;
f = 1000/180; % factor de conversión de g a mmol
 
% Comidas (perturbaciones) a lo largo de un día
if t >= 180*60 && t < 480*60 % ingesta de 75 g de HC
    t1 = 180*60;
    Dg = 50*f;
end
 
% Ecuación
D = (Dg*Ag*(t-t1)*exp(-(t-t1)/Tmaxi))/(Vg*Tmaxg^2);

== matlab function bergman_otro_modelo/Ingesta 75 g12 ==
  data: in input; D output
function D = comida(in)
% Variables de entrada en la funcion
t = in(1) %- 8*60*60; % Ajuste para iniciar a las 8 de la mañana
 
% Parámetros del modelo
Ag = 0.8; % adimensional
Tmaxi = 55*60; % s
Vg = 13.79; % L
Tmaxg = 40*60; % s
t1 = 0;
Dg = 0;
f = 1000/180; % factor de conversión de g a mmol
 
% Comidas (perturbaciones) a lo largo de un día
if t >= 180*60 && t < 480*60 % ingesta de 75 g de HC
    t1 = 180*60;
    Dg = 50*f;
end
 
% Ecuación
D = (Dg*Ag*(t-t1)*exp(-(t-t1)/Tmaxi))/(Vg*Tmaxg^2);

== matlab function bergman_otro_modelo/Ingesta 75 g13 ==
  data: in input; D output
function D = comida(in)
% Variables de entrada en la funcion
t = in(1) %- 8*60*60; % Ajuste para iniciar a las 8 de la mañana
 
% Parámetros del modelo
Ag = 0.8; % adimensional
Tmaxi = 55*60; % s
Vg = 13.79; % L
Tmaxg = 40*60; % s
t1 = 0;
Dg = 0;
f = 1000/180; % factor de conversión de g a mmol
 
% Comidas (perturbaciones) a lo largo de un día
if t >= 180*60 && t < 480*60 % ingesta de 75 g de HC
    t1 = 180*60;
    Dg = 50*f;
end
 
% Ecuación
D = (Dg*Ag*(t-t1)*exp(-(t-t1)/Tmaxi))/(Vg*Tmaxg^2);

== matlab function bergman_otro_modelo/Ingesta 75 g14 ==
  data: in input; D output
function D = comida(in)
% Variables de entrada en la funcion
t = in(1) %- 8*60*60; % Ajuste para iniciar a las 8 de la mañana
 
% Parámetros del modelo
Ag = 0.8; % adimensional
Tmaxi = 55*60; % s
Vg = 13.79; % L
Tmaxg = 40*60; % s
t1 = 0;
Dg = 0;
f = 1000/180; % factor de conversión de g a mmol
 
% Comidas (perturbaciones) a lo largo de un día
if t >= 180*60 && t < 480*60 % ingesta de 75 g de HC
    t1 = 180*60;
    Dg = 50*f;
end
 
% Ecuación
D = (Dg*Ag*(t-t1)*exp(-(t-t1)/Tmaxi))/(Vg*Tmaxg^2);

== matlab function bergman_otro_modelo/Ingesta 75 g15 ==
  data: in input; D output
function D = comida(in)
% Variables de entrada en la funcion
t = in(1) %- 8*60*60; % Ajuste para iniciar a las 8 de la mañana
 
% Parámetros del modelo
Ag = 0.8; % adimensional
Tmaxi = 55*60; % s
Vg = 13.79; % L
Tmaxg = 40*60; % s
t1 = 0;
Dg = 0;
f = 1000/180; % factor de conversión de g a mmol
 
% Comidas (perturbaciones) a lo largo de un día
if t >= 180*60 && t < 480*60 % ingesta de 75 g de HC
    t1 = 180*60;
    Dg = 50*f;
end
 
% Ecuación
D = (Dg*Ag*(t-t1)*exp(-(t-t1)/Tmaxi))/(Vg*Tmaxg^2);

== matlab function bergman_otro_modelo/Ingesta 75 g16 ==
  data: in input; D output
function D = comida(in)
% Variables de entrada en la funcion
t = in(1) %- 8*60*60; % Ajuste para iniciar a las 8 de la mañana
 
% Parámetros del modelo
Ag = 0.8; % adimensional
Tmaxi = 55*60; % s
Vg = 13.79; % L
Tmaxg = 40*60; % s
t1 = 0;
Dg = 0;
f = 1000/180; % factor de conversión de g a mmol
 
% Comidas (perturbaciones) a lo largo de un día
if t >= 180*60 && t < 480*60 % ingesta de 75 g de HC
    t1 = 180*60;
    Dg = 50*f;
end
 
% Ecuación
D = (Dg*Ag*(t-t1)*exp(-(t-t1)/Tmaxi))/(Vg*Tmaxg^2);

== matlab function bergman_otro_modelo/Ingesta 75 g8 ==
  data: in input; D output
function D = comida(in)
% Variables de entrada en la funcion
t = in(1) %- 8*60*60; % Ajuste para iniciar a las 8 de la mañana
 
% Parámetros del modelo
Ag = 0.8; % adimensional
Tmaxi = 55*60; % s
Vg = 13.79; % L
Tmaxg = 40*60; % s
t1 = 0;
Dg = 0;
f = 1000/180; % factor de conversión de g a mmol
 
% Comidas (perturbaciones) a lo largo de un día
if t >= 180*60 && t < 480*60 % ingesta de 75 g de HC
    t1 = 180*60;
    Dg = 50*f;
end
 
% Ecuación
D = (Dg*Ag*(t-t1)*exp(-(t-t1)/Tmaxi))/(Vg*Tmaxg^2);

== matlab function bergman_otro_modelo/Ingesta 75 g9 ==
  data: in input; D output
function D = comida(in)
% Variables de entrada en la funcion
t = in(1) %- 8*60*60; % Ajuste para iniciar a las 8 de la mañana
 
% Parámetros del modelo
Ag = 0.8; % adimensional
Tmaxi = 55*60; % s
Vg = 13.79; % L
Tmaxg = 40*60; % s
t1 = 0;
Dg = 0;
f = 1000/180; % factor de conversión de g a mmol
 
% Comidas (perturbaciones) a lo largo de un día
if t >= 180*60 && t < 480*60 % ingesta de 75 g de HC
    t1 = 180*60;
    Dg = 50*f;
end
 
% Ecuación
D = (Dg*Ag*(t-t1)*exp(-(t-t1)/Tmaxi))/(Vg*Tmaxg^2);

== matlab function bergman_otro_modelo/MATLAB Function10 ==
  data: in input; Ej output
function Ej  = ejercicio(in)
% Variables de entrada en la funcion
t = in(1);
%Parametros del modelo
cons = 0.005/60;
%Ejercicio (perturbaciones) a lo largo de un día

if t>=0 && t<60*60 %ejercicio 1 h
 Ej=0;
elseif t>=60*60 && t<180*60 %ejercicio 1 h
 Ej=cons+ 0.005/60;
else
 Ej=cons/2;
end

== matlab function bergman_otro_modelo/MATLAB Function11 ==
  data: in input; Ej output
function Ej  = ejercicio(in)
% Variables de entrada en la funcion
t = in(1);
%Parametros del modelo
cons = 0.005/60;
%Ejercicio (perturbaciones) a lo largo de un día

if t>=0 && t<240*60 %ejercicio 1 h
 Ej=0;
elseif t>=240*60 && t<360*60 %ejercicio 1 h
 Ej=cons+ 0.005/60;
else
 Ej=cons/2;
end

== matlab function bergman_otro_modelo/MATLAB Function12 ==
  data: in input; Ej output
function Ej  = ejercicio(in)
% Variables de entrada en la funcion
t = in(1);
%Parametros del modelo
cons = 0.005/60;
%Ejercicio (perturbaciones) a lo largo de un día

if t>=0 && t<240*60 %ejercicio 1 h
 Ej=0;
elseif t>=240*60 && t<360*60 %ejercicio 1 h
 Ej=cons+ 0.005/60;
else
 Ej=cons/2;
end

== matlab function bergman_otro_modelo/MATLAB Function7 ==
  data: in input; Ej output
function Ej  = ejercicio(in)
% Variables de entrada en la funcion
t = in(1);
%Parametros del modelo
cons = 0.005/60;
%Ejercicio (perturbaciones) a lo largo de un día

if t>=0 && t<240*60 %ejercicio 1 h
 Ej=0;
elseif t>=240*60 && t<360*60 %ejercicio 1 h
 Ej=cons+ 0.005/60;
else
 Ej=cons/2;
end

== matlab function bergman_otro_modelo/MATLAB Function8 ==
  data: in input; Ej output
function Ej  = ejercicio(in)
% Variables de entrada en la funcion
t = in(1);
%Parametros del modelo
cons = 0.005/60;
%Ejercicio (perturbaciones) a lo largo de un día

if t>=0 && t<240*60 %ejercicio 1 h
 Ej=0;
elseif t>=240*60 && t<360*60 %ejercicio 1 h
 Ej=cons+ 0.005/60;
else
 Ej=cons/2;
end

== matlab function bergman_otro_modelo/MATLAB Function9 ==
  data: in input; Ej output
function Ej  = ejercicio(in)
% Variables de entrada en la funcion
t = in(1);
%Parametros del modelo
cons = 0.005/60;
%Ejercicio (perturbaciones) a lo largo de un día

if t>=0 && t<240*60 %ejercicio 1 h
 Ej=0;
elseif t>=240*60 && t<360*60 %ejercicio 1 h
 Ej=cons+ 0.005/60;
else
 Ej=cons/2;
end
